simulink model "teste_controle"  (R2024b)
settings: Solver=VariableStepAuto  StartTime=0.0  StopTime=10.0  RelTol=1e-3
settings Model: Creator=henri  LastModifiedBy=henri

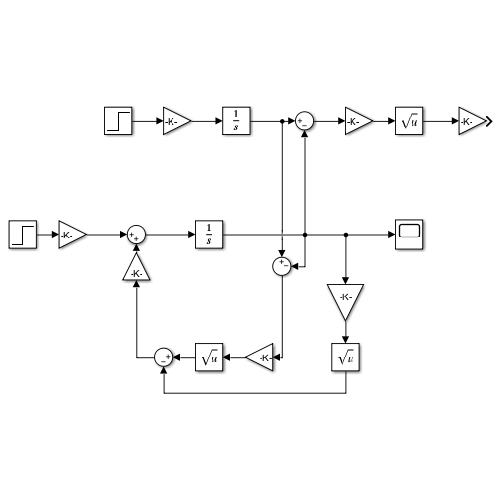
[thumbnail: Simulink's stored preview of the top-level diagram]
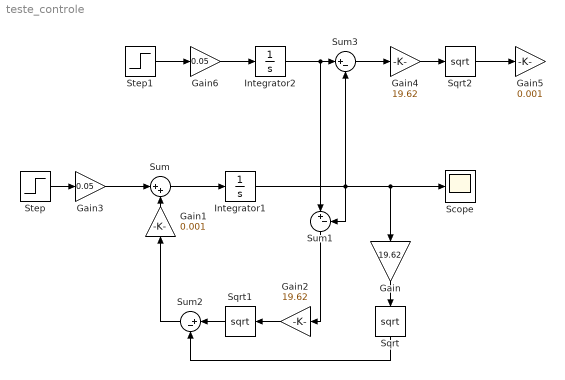
== system teste_controle ==
  Gain : Gain  Gain=19.62
  Gain1 : Gain  Gain=0.001
  Gain2 : Gain  Gain=19.62
  Gain3 : Gain  Gain=0.05
  Gain4 : Gain  Gain=19.62
  Gain5 : Gain  Gain=0.001
  Gain6 : Gain  Gain=0.05
  Integrator1 : Integrator
  Integrator2 : Integrator
  Scope : Scope
  Sqrt : Sqrt
  Sqrt1 : Sqrt
  Sqrt2 : Sqrt
  Step : Step  SampleTime=0
  Step1 : Step  SampleTime=0
  Sum : Sum  Inputs=|++
  Sum1 : Sum  Inputs=|+-
  Sum2 : Sum  Inputs=|+-
  Sum3 : Sum  Inputs=|+-
  wires:
  Integrator1/1 -> Scope/1, Gain/1, Sum3/2, Sum1/2
  Gain/1 -> Sqrt/1
  Sqrt/1 -> Sum2/2
  Gain2/1 -> Sqrt1/1
  Sqrt1/1 -> Sum2/1
  Sum/1 -> Integrator1/1
  Gain1/1 -> Sum/2
  Sum1/1 -> Gain2/1
  Sum2/1 -> Gain1/1
  Step/1 -> Gain3/1
  Gain3/1 -> Sum/1
  Integrator2/1 -> Sum1/1, Sum3/1
  Sum3/1 -> Gain4/1
  Gain4/1 -> Sqrt2/1
  Sqrt2/1 -> Gain5/1
  Gain6/1 -> Integrator2/1
  Step1/1 -> Gain6/1
